simulink library "Actuators"  (R2017b)
settings: Solver=VariableStepAuto  StartTime=0.0  StopTime=10.0  RelTol=1e-3
undefined symbols (not defined in the file or in its folder): r0, Rlim, Rmax, Rmin, Umax, Umin
libraries: dspmtrx3 x14, aerolibactuator x6, aerolibpropulsion2 x2
settings Model: Creator=Liam Uni  LastModifiedBy=Liam Uni

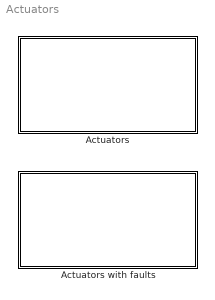
== system Actuators ==
  "Actuators " : Subsystem
      mask Display: disp('Actuators')
  Actuators with faults : Subsystem
      mask Display: disp('Actuators with Faults')

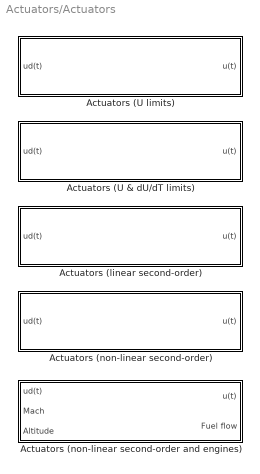
== system Actuators/Actuators  ==
  Actuators (U & dU/dT limits) : Subsystem  mask{Umax=Umax, Umin=Umin, u0=0, Rmax=Rmax, Rmin=Rmin, r0=r0}
      mask prompts: Umax "Max position"; Umin "Min position"; u0 "Initial position"; Rmax "Max rate"; Rmin "Min rate"; r0 "Initial rate"
      mask DialogControl DescGroupVar Prompt: Actuator Block
      mask DialogControl DescTextVar Prompt: Simple position and rate saturation blocks.
      mask DialogControl ParameterGroupVar Prompt: Position
      mask DialogControl Container3 Prompt: Rate
      mask Display:
      | port_label('input', 1, 'ud(t)');
      | 
      | port_label('output', 1, 'u(t)');
  Actuators (U limits) : Subsystem  mask{Umax=Umax, Umin=Umin, u0=0}
      mask prompts: Umax "Max position"; Umin "Min position"; u0 "Initial position"
      mask DialogControl DescGroupVar Prompt: Actuator Block
      mask DialogControl DescTextVar Prompt: Simple position saturation block.
      mask DialogControl ParameterGroupVar Prompt: Position
      mask Display:
      | port_label('input', 1, 'ud(t)');
      | 
      | port_label('output', 1, 'u(t)');
  Actuators (linear second-order) : Subsystem  mask{u0=0, r0=r0, omega=1, zeta=0.3}
      mask prompts: u0 "Initial position"; r0 "Initial rate"; omega "Natural frequency"; zeta "Damping ratio"
      mask DialogControl DescGroupVar Prompt: Actuator Block
      mask DialogControl DescTextVar Prompt: Linear second-order dynamic actuators.
      mask DialogControl ParameterGroupVar Prompt: Position
      mask DialogControl Container3 Prompt: Rate
      mask DialogControl Container4 Prompt: Dynamics
      mask Display:
      | port_label('input', 1, 'ud(t)');
      | 
      | port_label('output', 1, 'u(t)');
  Actuators (non-linear second-order and engines) : Subsystem  mask{Umax=Umax, Umin=Umin, u0=0, Rlim=Rlim, r0=r0, omega=1, zeta=0.3, E=3, Parameter8=0, TMax=45000, Te=1, Tsf=0.35, Tr=0.9}
      mask prompts: Umax "Max position"; Umin "Min position"; u0 "Initial position"; Rlim "Rate limit"; r0 "Initial rate"; omega "Natural frequency"; zeta "Damping ratio"; E "Number of engines"; Parameter8 "Initial thrust"; TMax "Max sea-level static thrust"; Te "Fastest engine time constant at sea-level static"; Tsf "Sea-level static thrust specific fuel consumption"; Tr "Ratio of installed thrust to uninstalled thrust"
      mask DialogControl DescGroupVar Prompt: Actuator Block
      mask DialogControl DescTextVar Prompt: Non-linear second-order dynamic actuators and first-order engines.
      mask DialogControl Container6 Prompt: Actuators
      mask DialogControl ParameterGroupVar Prompt: Position
      mask DialogControl Container3 Prompt: Rate
      mask DialogControl Container4 Prompt: Dynamics
      mask DialogControl Container9 Prompt: Engines
      mask Display:
      | port_label('input', 1, 'ud(t)');
      | port_label('input', 2, 'Mach');
      | port_label('input', 3, 'Altitude');
      | port_label('output', 1, 'u(t)');
      | port_label('output', 2, 'Fuel flow');
  Actuators (non-linear second-order) : Subsystem  mask{Umax=Umax, Umin=Umin, u0=0, Rlim=Rlim, r0=r0, omega=1, zeta=0.3}
      mask prompts: Umax "Max position"; Umin "Min position"; u0 "Initial position"; Rlim "Rate limit"; r0 "Initial rate"; omega "Natural frequency"; zeta "Damping ratio"
      mask DialogControl DescGroupVar Prompt: Actuator Block
      mask DialogControl DescTextVar Prompt: Non-linear second-order dynamic actuators.
      mask DialogControl ParameterGroupVar Prompt: Position
      mask DialogControl Container3 Prompt: Rate
      mask DialogControl Container4 Prompt: Dynamics
      mask Display:
      | port_label('input', 1, 'ud(t)');
      | 
      | port_label('output', 1, 'u(t)');

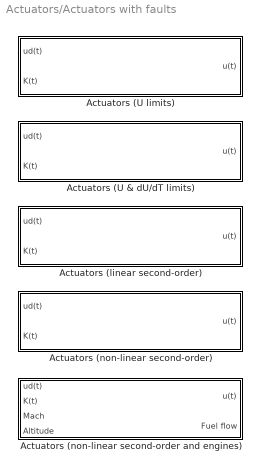
== system Actuators/Actuators with faults ==
  Actuators (U & dU/dT limits) : Subsystem  mask{Umax=Umax, Umin=Umin, u0=0, Rmax=Rmax, Rmin=Rmin, r0=r0}
      mask prompts: Umax "Max position"; Umin "Min position"; u0 "Initial position"; Rmax "Max rate"; Rmin "Min rate"; r0 "Initial rate"
      mask DialogControl DescGroupVar Prompt: Actuator Block
      mask DialogControl DescTextVar Prompt: Simple position and rate saturation blocks with an effectiveness fault.
      mask DialogControl ParameterGroupVar Prompt: Position
      mask DialogControl Container3 Prompt: Rate
      mask Display:
      | port_label('input', 1, 'ud(t)');
      | port_label('input', 2, 'K(t)');
      | port_label('output', 1, 'u(t)');
  Actuators (U limits) : Subsystem  mask{Umax=Umax, Umin=Umin, u0=0}
      mask prompts: Umax "Max position"; Umin "Min position"; u0 "Initial position"
      mask DialogControl DescGroupVar Prompt: Actuator Block
      mask DialogControl DescTextVar Prompt: Simple position saturation block with an effectiveness fault.
      mask DialogControl ParameterGroupVar Prompt: Position
      mask Display:
      | port_label('input', 1, 'ud(t)');
      | port_label('input', 2, 'K(t)');
      | port_label('output', 1, 'u(t)');
  Actuators (linear second-order) : Subsystem  mask{u0=0, r0=r0, omega=1, zeta=0.3}
      mask prompts: u0 "Initial position"; r0 "Initial rate"; omega "Natural frequency"; zeta "Damping ratio"
      mask DialogControl DescGroupVar Prompt: Actuator Block
      mask DialogControl DescTextVar Prompt: Linear second-order dynamic actuators with an effectiveness fault.
      mask DialogControl ParameterGroupVar Prompt: Position
      mask DialogControl Container3 Prompt: Rate
      mask DialogControl Container4 Prompt: Dynamics
      mask Display:
      | port_label('input', 1, 'ud(t)');
      | port_label('input', 2, 'K(t)');
      | port_label('output', 1, 'u(t)');
  Actuators (non-linear second-order and engines) : Subsystem  mask{Umax=Umax, Umin=Umin, u0=0, Rlim=Rlim, r0=r0, omega=1, zeta=0.3, E=3, Parameter8=0, TMax=45000, Te=1, Tsf=0.35, Tr=0.9}
      mask prompts: Umax "Max position"; Umin "Min position"; u0 "Initial position"; Rlim "Rate limit"; r0 "Initial rate"; omega "Natural frequency"; zeta "Damping ratio"; E "Number of engines"; Parameter8 "Initial thrust"; TMax "Max sea-level static thrust"; Te "Fastest engine time constant at sea-level static"; Tsf "Sea-level static thrust specific fuel consumption"; Tr "Ratio of installed thrust to uninstalled thrust"
      mask DialogControl DescGroupVar Prompt: Actuator Block
      mask DialogControl DescTextVar Prompt: Non-linear second-order dynamic actuators and first-order engines, with an effectiveness fault.
      mask DialogControl Container6 Prompt: Actuators
      mask DialogControl ParameterGroupVar Prompt: Position
      mask DialogControl Container3 Prompt: Rate
      mask DialogControl Container4 Prompt: Dynamics
      mask DialogControl Container9 Prompt: Engines
      mask Display:
      | port_label('input', 1, 'ud(t)');
      | port_label('input', 2, 'K(t)');
      | port_label('input', 3, 'Mach');
      | port_label('input', 4, 'Altitude');
      | port_label('output', 1, 'u(t)');
      | port_label('output', 2, 'Fuel flow');
  Actuators (non-linear second-order) : Subsystem  mask{Umax=Umax, Umin=Umin, u0=0, Rlim=Rlim, r0=r0, omega=1, zeta=0.3}
      mask prompts: Umax "Max position"; Umin "Min position"; u0 "Initial position"; Rlim "Rate limit"; r0 "Initial rate"; omega "Natural frequency"; zeta "Damping ratio"
      mask DialogControl DescGroupVar Prompt: Actuator Block
      mask DialogControl DescTextVar Prompt: Non-linear second-order dynamic actuators with an effectiveness fault.
      mask DialogControl ParameterGroupVar Prompt: Position
      mask DialogControl Container3 Prompt: Rate
      mask DialogControl Container4 Prompt: Dynamics
      mask Display:
      | port_label('input', 1, 'ud(t)');
      | port_label('input', 2, 'K(t)');
      | port_label('output', 1, 'u(t)');

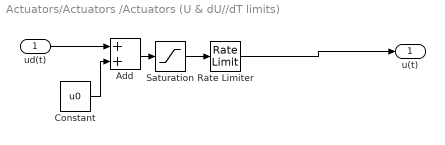
== system Actuators/Actuators /Actuators (U & dU//dT limits) ==
  ud(t) : Inport
  Add : Sum
  Constant : Constant  Value=u0
  Rate Limiter : RateLimiter  RisingSlewLimit=Rmax  FallingSlewLimit=Rmin  SampleTimeMode=inherited  InitialCondition=r0
  Saturation : Saturate  UpperLimit=Umax  LowerLimit=Umin
  u(t) : Outport
  wires:
  ud(t)/1 -> Add/1
  Saturation/1 -> Rate Limiter/1
  Rate Limiter/1 -> u(t)/1
  Add/1 -> Saturation/1
  Constant/1 -> Add/2

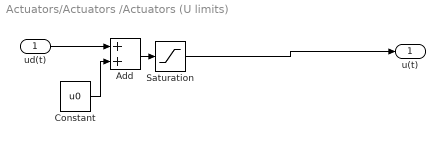
== system Actuators/Actuators /Actuators (U limits) ==
  ud(t) : Inport
  Add : Sum
  Constant : Constant  Value=u0
  Saturation : Saturate  UpperLimit=Umax  LowerLimit=Umin
  u(t) : Outport
  wires:
  ud(t)/1 -> Add/1
  Saturation/1 -> u(t)/1
  Add/1 -> Saturation/1
  Constant/1 -> Add/2

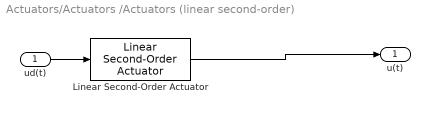
== system Actuators/Actuators /Actuators (linear second-order) ==
  ud(t) : Inport
  Linear Second-Order Actuator : aerolibactuator/Linear Second-Order Actuator  wn_fin=omega  z_fin=zeta  fin_act_0=u0  fin_act_vel=r0
      settings: SourceProductName=Aerospace Blockset  SourceProductBaseCode=AE
  u(t) : Outport
  wires:
  Linear Second-Order Actuator/1 -> u(t)/1
  ud(t)/1 -> Linear Second-Order Actuator/1

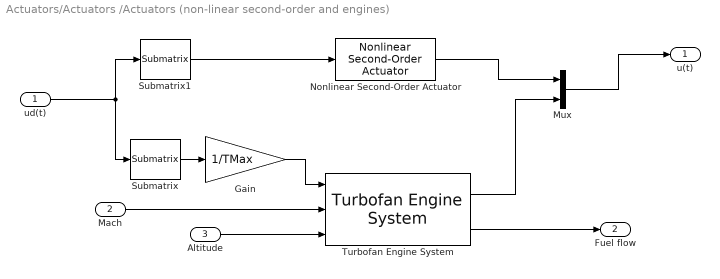
== system Actuators/Actuators /Actuators (non-linear second-order and engines) ==
  ud(t) : Inport
  Mach : Inport  Port=2
  Altitude : Inport  Port=3
  Gain : Gain  Gain=1/TMax
  Mux : Mux  Inputs=2
  Nonlinear Second-Order Actuator : aerolibactuator/Nonlinear Second-Order Actuator  wn_fin=omega  z_fin=zeta  fin_max=Umax  fin_min=Umin  fin_maxrate=Rlim  fin_act_0=u0  fin_act_vel=r0
      settings: SourceProductName=Aerospace Blockset  SourceProductBaseCode=AE
  Submatrix : dspmtrx3/Submatrix  RowSpan=Range of rows  RowStartMode=Offset from last  RowStartIndex=E-1  RowEndMode=Last  RowEndIndex=1  ColSpan=Range of columns  ColStartMode=First  ColStartIndex=1  ColEndMode=Last  ColEndIndex=1
  Submatrix1 : dspmtrx3/Submatrix  RowSpan=Range of rows  RowStartMode=First  RowStartIndex=E-1  RowEndMode=Offset from last  RowEndIndex=E  ColSpan=Range of columns  ColStartMode=First  ColStartIndex=1  ColEndMode=Last  ColEndIndex=1
  Turbofan Engine System : aerolibpropulsion2/Turbofan Engine System  units=Metric (MKS)  ic_source=Internal  IC=T0  Fmax=TMax  tau=Te  SFC=Tsf  Nt=Tr
      settings: SourceProductName=Aerospace Blockset  SourceProductBaseCode=AE
  u(t) : Outport
  Fuel flow : Outport  Port=2
  wires:
  ud(t)/1 -> Submatrix/1, Submatrix1/1
  Nonlinear Second-Order Actuator/1 -> Mux/1
  Mux/1 -> u(t)/1
  Submatrix/1 -> Gain/1
  Submatrix1/1 -> Nonlinear Second-Order Actuator/1
  Gain/1 -> Turbofan Engine System/1
  Mach/1 -> Turbofan Engine System/2
  Altitude/1 -> Turbofan Engine System/3
  Turbofan Engine System/1 -> Mux/2
  Turbofan Engine System/2 -> Fuel flow/1

== system Actuators/Actuators /Actuators (non-linear second-order) ==
  ud(t) : Inport
  Nonlinear Second-Order Actuator : aerolibactuator/Nonlinear Second-Order Actuator  wn_fin=omega  z_fin=zeta  fin_max=Umax  fin_min=Umin  fin_maxrate=Rlim  fin_act_0=u0  fin_act_vel=r0
      settings: SourceProductName=Aerospace Blockset  SourceProductBaseCode=AE
  u(t) : Outport
  wires:
  Nonlinear Second-Order Actuator/1 -> u(t)/1
  ud(t)/1 -> Nonlinear Second-Order Actuator/1

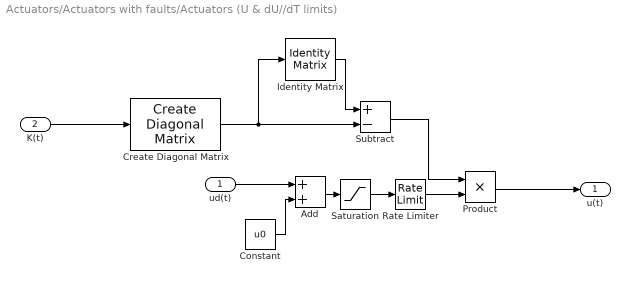
== system Actuators/Actuators with faults/Actuators (U & dU//dT limits) ==
  ud(t) : Inport
  K(t) : Inport  Port=2
  Add : Sum
  Constant : Constant  Value=u0
  Create Diagonal Matrix : dspmtrx3/Create Diagonal Matrix
      settings: SourceProductName=DSP System Toolbox  SourceProductBaseCode=DS
  Identity Matrix : dspmtrx3/Identity Matrix  Inherit=on  N=5  Ts=1  dataType=double  isSigned=on  wordLen=16  udDataType=sfix(16)  fracBitsMode=Best precision  numFracBits=15  OutDataTypeStr=double  LastOutDataTypeStr=double
      settings: SourceProductName=DSP System Toolbox
  Product : Product
  Rate Limiter : RateLimiter  RisingSlewLimit=Rmax  FallingSlewLimit=Rmin  SampleTimeMode=inherited  InitialCondition=r0
  Saturation : Saturate  UpperLimit=Umax  LowerLimit=Umin
  Subtract : Sum  Inputs=+-
  u(t) : Outport
  wires:
  ud(t)/1 -> Add/1
  Saturation/1 -> Rate Limiter/1
  Product/1 -> u(t)/1
  Create Diagonal Matrix/1 -> Identity Matrix/1, Subtract/2
  K(t)/1 -> Create Diagonal Matrix/1
  Identity Matrix/1 -> Subtract/1
  Subtract/1 -> Product/1
  Add/1 -> Saturation/1
  Constant/1 -> Add/2
  Rate Limiter/1 -> Product/2

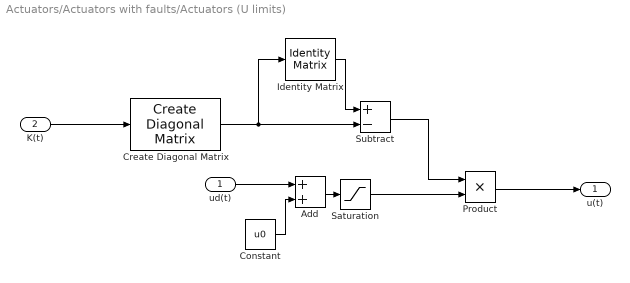
== system Actuators/Actuators with faults/Actuators (U limits) ==
  ud(t) : Inport
  K(t) : Inport  Port=2
  Add : Sum
  Constant : Constant  Value=u0
  Create Diagonal Matrix : dspmtrx3/Create Diagonal Matrix
      settings: SourceProductName=DSP System Toolbox  SourceProductBaseCode=DS
  Identity Matrix : dspmtrx3/Identity Matrix  Inherit=on  N=5  Ts=1  dataType=double  isSigned=on  wordLen=16  udDataType=sfix(16)  fracBitsMode=Best precision  numFracBits=15  OutDataTypeStr=double  LastOutDataTypeStr=double
      settings: SourceProductName=DSP System Toolbox
  Product : Product
  Saturation : Saturate  UpperLimit=Umax  LowerLimit=Umin
  Subtract : Sum  Inputs=+-
  u(t) : Outport
  wires:
  ud(t)/1 -> Add/1
  Saturation/1 -> Product/2
  Product/1 -> u(t)/1
  Create Diagonal Matrix/1 -> Identity Matrix/1, Subtract/2
  K(t)/1 -> Create Diagonal Matrix/1
  Identity Matrix/1 -> Subtract/1
  Subtract/1 -> Product/1
  Add/1 -> Saturation/1
  Constant/1 -> Add/2

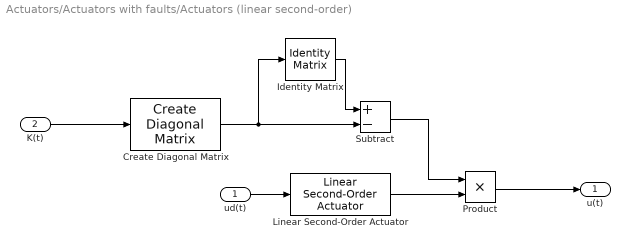
== system Actuators/Actuators with faults/Actuators (linear second-order) ==
  ud(t) : Inport
  K(t) : Inport  Port=2
  Create Diagonal Matrix : dspmtrx3/Create Diagonal Matrix
      settings: SourceProductName=DSP System Toolbox  SourceProductBaseCode=DS
  Identity Matrix : dspmtrx3/Identity Matrix  Inherit=on  N=5  Ts=1  dataType=double  isSigned=on  wordLen=16  udDataType=sfix(16)  fracBitsMode=Best precision  numFracBits=15  OutDataTypeStr=double  LastOutDataTypeStr=double
      settings: SourceProductName=DSP System Toolbox
  Linear Second-Order Actuator : aerolibactuator/Linear Second-Order Actuator  wn_fin=omega  z_fin=zeta  fin_act_0=u0  fin_act_vel=r0
      settings: SourceProductName=Aerospace Blockset  SourceProductBaseCode=AE
  Product : Product
  Subtract : Sum  Inputs=+-
  u(t) : Outport
  wires:
  Product/1 -> u(t)/1
  Create Diagonal Matrix/1 -> Identity Matrix/1, Subtract/2
  K(t)/1 -> Create Diagonal Matrix/1
  Identity Matrix/1 -> Subtract/1
  Subtract/1 -> Product/1
  Linear Second-Order Actuator/1 -> Product/2
  ud(t)/1 -> Linear Second-Order Actuator/1

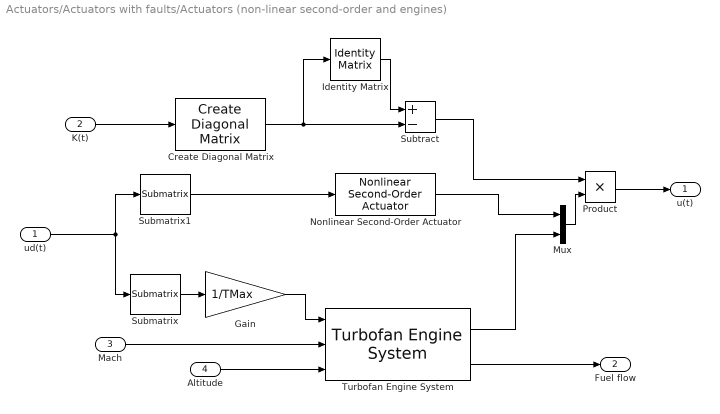
== system Actuators/Actuators with faults/Actuators (non-linear second-order and engines) ==
  ud(t) : Inport
  K(t) : Inport  Port=2
  Mach : Inport  Port=3
  Altitude : Inport  Port=4
  Create Diagonal Matrix : dspmtrx3/Create Diagonal Matrix
      settings: SourceProductName=DSP System Toolbox  SourceProductBaseCode=DS
  Gain : Gain  Gain=1/TMax
  Identity Matrix : dspmtrx3/Identity Matrix  Inherit=on  N=5  Ts=1  dataType=double  isSigned=on  wordLen=16  udDataType=sfix(16)  fracBitsMode=Best precision  numFracBits=15  OutDataTypeStr=double  LastOutDataTypeStr=double
      settings: SourceProductName=DSP System Toolbox
  Mux : Mux  Inputs=2
  Nonlinear Second-Order Actuator : aerolibactuator/Nonlinear Second-Order Actuator  wn_fin=omega  z_fin=zeta  fin_max=Umax  fin_min=Umin  fin_maxrate=Rlim  fin_act_0=u0  fin_act_vel=r0
      settings: SourceProductName=Aerospace Blockset  SourceProductBaseCode=AE
  Product : Product
  Submatrix : dspmtrx3/Submatrix  RowSpan=Range of rows  RowStartMode=Offset from last  RowStartIndex=E-1  RowEndMode=Last  RowEndIndex=1  ColSpan=Range of columns  ColStartMode=First  ColStartIndex=1  ColEndMode=Last  ColEndIndex=1
  Submatrix1 : dspmtrx3/Submatrix  RowSpan=Range of rows  RowStartMode=First  RowStartIndex=E-1  RowEndMode=Offset from last  RowEndIndex=E  ColSpan=Range of columns  ColStartMode=First  ColStartIndex=1  ColEndMode=Last  ColEndIndex=1
  Subtract : Sum  Inputs=+-
  Turbofan Engine System : aerolibpropulsion2/Turbofan Engine System  units=Metric (MKS)  ic_source=Internal  IC=T0  Fmax=TMax  tau=Te  SFC=Tsf  Nt=Tr
      settings: SourceProductName=Aerospace Blockset  SourceProductBaseCode=AE
  u(t) : Outport
  Fuel flow : Outport  Port=2
  wires:
  ud(t)/1 -> Submatrix/1, Submatrix1/1
  Nonlinear Second-Order Actuator/1 -> Mux/1
  Subtract/1 -> Product/1
  Identity Matrix/1 -> Subtract/1
  K(t)/1 -> Create Diagonal Matrix/1
  Create Diagonal Matrix/1 -> Subtract/2, Identity Matrix/1
  Product/1 -> u(t)/1
  Submatrix/1 -> Gain/1
  Submatrix1/1 -> Nonlinear Second-Order Actuator/1
  Gain/1 -> Turbofan Engine System/1
  Mach/1 -> Turbofan Engine System/2
  Altitude/1 -> Turbofan Engine System/3
  Turbofan Engine System/1 -> Mux/2
  Mux/1 -> Product/2
  Turbofan Engine System/2 -> Fuel flow/1

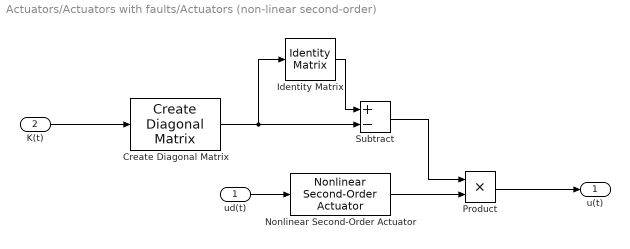
== system Actuators/Actuators with faults/Actuators (non-linear second-order) ==
  ud(t) : Inport
  K(t) : Inport  Port=2
  Create Diagonal Matrix : dspmtrx3/Create Diagonal Matrix
      settings: SourceProductName=DSP System Toolbox  SourceProductBaseCode=DS
  Identity Matrix : dspmtrx3/Identity Matrix  Inherit=on  N=5  Ts=1  dataType=double  isSigned=on  wordLen=16  udDataType=sfix(16)  fracBitsMode=Best precision  numFracBits=15  OutDataTypeStr=double  LastOutDataTypeStr=double
      settings: SourceProductName=DSP System Toolbox
  Nonlinear Second-Order Actuator : aerolibactuator/Nonlinear Second-Order Actuator  wn_fin=omega  z_fin=zeta  fin_max=Umax  fin_min=Umin  fin_maxrate=Rlim  fin_act_0=u0  fin_act_vel=r0
      settings: SourceProductName=Aerospace Blockset  SourceProductBaseCode=AE
  Product : Product
  Subtract : Sum  Inputs=+-
  u(t) : Outport
  wires:
  Product/1 -> u(t)/1
  Create Diagonal Matrix/1 -> Identity Matrix/1, Subtract/2
  K(t)/1 -> Create Diagonal Matrix/1
  Identity Matrix/1 -> Subtract/1
  Subtract/1 -> Product/1
  Nonlinear Second-Order Actuator/1 -> Product/2
  ud(t)/1 -> Nonlinear Second-Order Actuator/1
